simulink model "SBW_PID_controller"  (R2024b)
settings: Solver=FixedStepAuto  StartTime=0.0  StopTime=inf  FixedStep=0.001  RelTol=1e-3
model workspace (MAT data in the model file):
  th = 1
libraries: arduinolib x14, simulink x5, slpidlib x2
settings Model: ExtModeTrigDuration=2  Creator=masas  LastModifiedBy=masas
settings SolverCC: AutoInsertRateTranBlk=on
settings OptimizationCC: EnhancedBackFolding=on  PassReuseOutputArgsAs=Individual arguments  ZeroExternalMemoryAtStartup=off  ZeroInternalMemoryAtStartup=off  MaxStackSize=64  OptimizeBlockOrder=speed  DifferentSizesBufferReuse=on  OptimizationCustomize=off  EfficientTunableParamExpr=on
settings DebuggingCC: ParameterTunabilityLossMsg=error
settings HardwareCC: ProdBitPerInt=16  ProdBitPerPointer=16  ProdBitPerSizeT=16  ProdBitPerPtrDiffT=16  ProdLargestAtomicFloat=None  ProdWordSize=8  ProdHWDeviceType=Atmel->AVR  UseEmbeddedCoderFeatures=off
settings SFSimCC: MATLABDynamicMemAlloc=off
settings RTWCC: Description=Embedded Coder  SystemTargetFile=ert.tlc  HardwareBoard=Arduino Uno  TemplateMakefile=ert_default_tmf  Toolchain=Arduino AVR  BuildConfiguration=Faster Runs
settings CodeAppCC: ForceParamTrailComments=on  IgnoreCustomStorageClasses=off  OperatorAnnotations=on  SimulinkDataObjDesc=on  SFDataObjDesc=on  InsertBlockDesc=on
settings ERTTargetCC: SupportContinuousTime=on  SupportNonInlinedSFcns=on  SupportVariableSizeSignals=on  ExtModeTransport=3  ExtModeStaticAlloc=on  ExtModeAutomaticAllocSize=off  ExtModeStaticAllocSize=250  ExtModeMexFile=ext_xcp  ExtModeIntrfLevel=Level2 - Open  InlinedParameterPlacement=Hierarchical

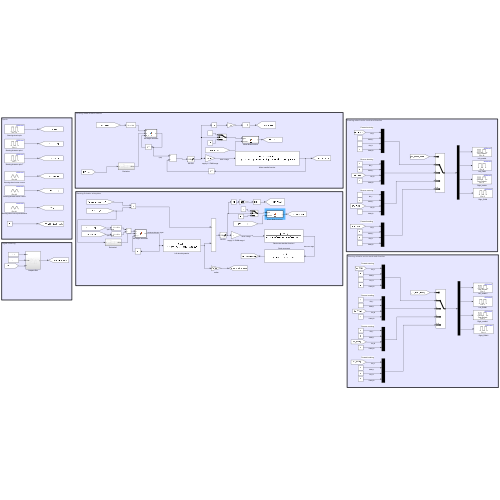
[thumbnail: Simulink's stored preview of the top-level diagram]
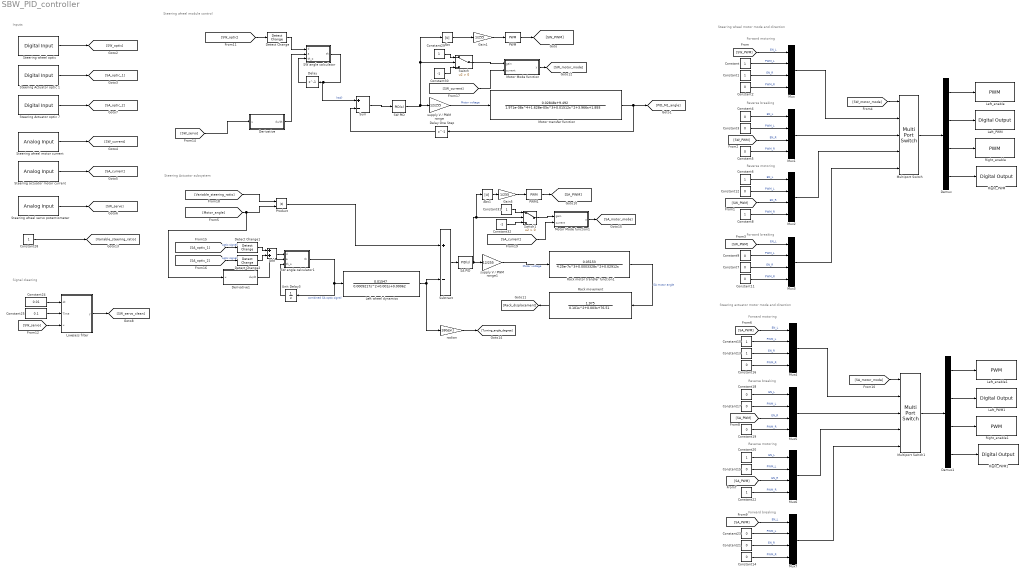
== system SBW_PID_controller ==
  note: Steering Actuator subsystem
  note: Signal cleaning
  note: Inputs
  note: Steering wheel module control
  note: Forward motoring
  note: Steering wheel motor mode and direction
  note: Reverse breaking
  note: Reverse motoring
  note: Forward breaking
  note: Forward breaking
  note: Reverse motoring
  note: Steering actuator motor mode and direction
  note: Forward motoring
  note: Reverse breaking
  Abs : Abs  SaturateOnIntegerOverflow=off
  Abs1 : Abs  SaturateOnIntegerOverflow=off
  Add : Sum
  Constant{,1,6,8,10,13,20,22,28..29,31} (11 alike) : Constant
  Constant{2..5,7,9,11..12,14..19,21,23} (16 alike) : Constant  Value=0
  Constant24 : Constant  Value=0.01
  Constant25 : Constant  Value=0.1
  Constant30 : Constant  Value=-1
  Constant32 : Constant  Value=-1
  Delay : Delay  DelayLength=1
  Delay One Step : Delay  DelayLength=1
  Demux : Demux
  Demux1 : Demux
  Derivative : Subsystem
  Derivative1 : Subsystem
  Detect Change : simulink/Logic and Bit Operations/Detect Change  vinit=0  OutDataTypeStr=boolean
  Detect Change1 : simulink/Logic and Bit Operations/Detect Change  vinit=0  OutDataTypeStr=boolean
  Detect Change2 : simulink/Logic and Bit Operations/Detect Change  vinit=0  OutDataTypeStr=boolean
  Gain1 : Gain  Gain=1/255
  Gain5 : Gain  Gain=1/255
  Left wheel dynamics : TransferFcn  Numerator=[0.01547]  Denominator=[0.0009217 0.001 0.00062]
  Left_PWM : arduinolib/Digital Output  pinNumber=8  Direction=output  blockPlatform=arduino
      settings: SourceProductName=Common
  Left_PWM1 : arduinolib/Digital Output  pinNumber=3  Direction=output  blockPlatform=arduino
      settings: SourceProductName=Common
  Left_enable : arduinolib/PWM  pinNumber=10  frequencyType=Default  desiredFrequency=490.2  achievableFrequency=490.2
      settings: SourceProductName=Common
  Left_enable1 : arduinolib/PWM  pinNumber=5  frequencyType=Default  desiredFrequency=490.2  achievableFrequency=490.2
      settings: SourceProductName=Common
  Lowpass filter : Subsystem
  Motor Mode function : MATLAB Function  TreatAsAtomicUnit=on
  Motor Mode function1 : MATLAB Function  TreatAsAtomicUnit=on
  Motor transfer function : TransferFcn  Numerator=[0.02848 9.492]  Denominator=|
      | [1.971e-08 1.628e-05 0.01512  3.966 1.893
      |  ]
  Multiport Switch : MultiPortSwitch  Inputs=4  SaturateOnIntegerOverflow=off  InputSameDT=off
  Multiport Switch1 : MultiPortSwitch  Inputs=4  SaturateOnIntegerOverflow=off  InputSameDT=off
  Mux{,1..7} (8 alike) : Mux
  PWM : simulink/Discontinuities/PWM  DisableCoverage=on  Period=0.01  InitialDelay=0  DisallowZeroDutyCycle=off  RunAtFixedTimeIntervals=on  SampleTime=0.1
  PWM1 : simulink/Discontinuities/PWM  DisableCoverage=on  Period=0.01  InitialDelay=0  DisallowZeroDutyCycle=off  RunAtFixedTimeIntervals=on  SampleTime=0.1
  Product : Product
  Rack motor transfer function1 : TransferFcn  Numerator=[0.05153]  Denominator=[4.25e-7 0.0003328 0.02912 0]
  Rack movement : TransferFcn  Numerator=[1.975]  Denominator=[0.101 0.003 76.51]
  Right_PWM : arduinolib/Digital Output  pinNumber=9  Direction=output  blockPlatform=arduino
      settings: SourceProductName=Common
  Right_PWM1 : arduinolib/Digital Output  pinNumber=4  Direction=output  blockPlatform=arduino
      settings: SourceProductName=Common
  Right_enable : arduinolib/PWM  pinNumber=11  frequencyType=Default  desiredFrequency=490.2  achievableFrequency=490.2
      settings: SourceProductName=Common
  Right_enable1 : arduinolib/PWM  pinNumber=6  frequencyType=Default  desiredFrequency=490.2  achievableFrequency=490.2
      settings: SourceProductName=Common
  "SA PID " : slpidlib/PID Controller  Controller=PID  Form=Parallel  TimeDomain=Continuous-time  UseExternalTs=off  SampleTime=-1  IntegratorMethod=Forward Euler  FilterMethod=Forward Euler  ControllerParametersSource=internal  P=6.187  I=0.03716  UseKiTs=off  D=19.07  UseExternalDerivativeSource=off  N=7.338  UseFilter=on  TunerSelectOption=Transfer Function Based (PID Tuner App)  InitialConditionSource=internal  InitialConditionForIntegrator=0  InitialConditionForFilter=0  DifferentiatorICPrevScaledInput=0  ExternalReset=none  TrackingMode=off  Kt=1  LimitOutput=on  SatLimitsSource=internal  UpperSaturationLimit=255  LowerSaturationLimit=-255  LinearizeAsGain=on  AntiWindupMode=none  Kb=1  LimitIntegrator=off  UpperIntegratorSaturationLimit=inf  LowerIntegratorSaturationLimit=-inf  POutMin=[]  POutMax=[]  IOutMin=[]  IOutMax=[]  DOutMin=[]  DOutMax=[]  NOutMin=[]  NOutMax=[]  SumOutMin=[]  SumOutMax=[]  SaturationOutMin=[]  SaturationOutMax=[]  PParamMin=[]  PParamMax=[]  IParamMin=[]  IParamMax=[]  DParamMin=[]  DParamMax=[]  NParamMin=[]  NParamMax=[]  KbParamMin=[]  KbParamMax=[]  KtParamMin=[]  KtParamMax=[]  KbOutMin=[]  KbOutMax=[]  KtOutMin=[]  KtOutMax=[]  IntegratorOutMin=[]  IntegratorOutMax=[]  FilterOutMin=[]  FilterOutMax=[]  SumI1OutMin=[]  SumI1OutMax=[]  SumI2OutMin=[]  SumI2OutMax=[]  SumI3OutMin=[]  SumI3OutMax=[]  SumI4OutMin=[]  SumI4OutMax=[]  SumDOutMin=[]  SumDOutMax=[]  DifferentiatorOutMin=[]  DifferentiatorOutMax=[]  FilterDiffOutCoefMin=[]  FilterDiffOutCoefMax=[]  ReciprocalOutMin=[]  ReciprocalOutMax=[]  SumDenOutMin=[]  SumDenOutMax=[]  SumNumOutMin=[]  SumNumOutMax=[]  DivideOutMin=[]  DivideOutMax=[]  UdiffTsProdOutMin=[]  UdiffTsProdOutMax=[]  NTsProdOutMin=[]  NTsProdOutMax=[]  UintegralTsProdOutMin=[]  UintegralTsProdOutMax=[]  UngainTsProdOutMin=[]  UngainTsProdOutMax=[]  ClampingZeroOutDataTypeStr=Inherit: Inherit via back propagation  ClampingZeroOutMin=[]  ClampingZeroOutMax=[]  FilterDenConstantOutDataTypeStr=Inherit: Inherit via back propagation  FilterDenConstantOutMin=[]  FilterDenConstantOutMax=[]  PCopyOutDataTypeStr=Inherit: Inherit via back propagation  PCopyOutMin=[]  PCopyOutMax=[]  NCopyOutDataTypeStr=Inherit: Inherit via back propagation  NCopyOutMin=[]  NCopyOutMax=[]  IntegratorContinuousStateAttributes=''  IntegratorStateMustResolveToSignalObject=off  IntegratorRTWStateStorageClass=Auto  FilterContinuousStateAttributes=''  FilterStateMustResolveToSignalObject=off  FilterRTWStateStorageClass=Auto  ParallelPVariant=InternalParameters  IdealPVariant=Disabled  IVariant=InternalParameters  DVariant=InternalParameters  IntegratorVariant=Continuous  SatVariant=Enabled  AWVariant=Passthrough  PCopyVariant=Disabled  TRVariant=Disabled  FdbkBlocksVariant=Forward  IdealPFdbkVariant=Disabled  SatFdbkVariant=Disabled  DerivativeFilterVariant=ContFilter  NVariant=InternalParameters  NCopyVariant=Disabled  FilterICVariant=InternalICsFilter  IntegratorICVariant=InternalICs  ExternalResetVariant=Disabled  TRSumVariant=Passthrough  SumFdbkVariant=Disabled  SumVariant=Sum_PID  TsampFilterVariant=InternalTs  TsampNgainVariant=Passthrough  TsampIntegralVariant=Disabled_SignalSpec  ExternalSaturationOutDataTypeStr=Inherit: Same as second input  DerivativeSourceVariant=ErrorSignal  PreIntVariant=InternalPreInt
  SW PID : slpidlib/PID Controller  Controller=PID  Form=Parallel  TimeDomain=Continuous-time  UseExternalTs=off  SampleTime=-1  IntegratorMethod=Forward Euler  FilterMethod=Forward Euler  ControllerParametersSource=internal  P=11.4731917903182  I=4.9291893088192  UseKiTs=off  D=3.34423646974898  UseExternalDerivativeSource=off  N=2.10860492250304  UseFilter=on  TunerSelectOption=Transfer Function Based (PID Tuner App)  InitialConditionSource=internal  InitialConditionForIntegrator=0  InitialConditionForFilter=0  DifferentiatorICPrevScaledInput=0  ExternalReset=none  TrackingMode=off  Kt=1  LimitOutput=on  SatLimitsSource=internal  UpperSaturationLimit=255  LowerSaturationLimit=-255  LinearizeAsGain=on  AntiWindupMode=clamping  Kb=1  LimitIntegrator=off  UpperIntegratorSaturationLimit=inf  LowerIntegratorSaturationLimit=-inf  POutMin=[]  POutMax=[]  IOutMin=[]  IOutMax=[]  DOutMin=[]  DOutMax=[]  NOutMin=[]  NOutMax=[]  SumOutMin=[]  SumOutMax=[]  SaturationOutMin=[]  SaturationOutMax=[]  PParamMin=[]  PParamMax=[]  IParamMin=[]  IParamMax=[]  DParamMin=[]  DParamMax=[]  NParamMin=[]  NParamMax=[]  KbParamMin=[]  KbParamMax=[]  KtParamMin=[]  KtParamMax=[]  KbOutMin=[]  KbOutMax=[]  KtOutMin=[]  KtOutMax=[]  IntegratorOutMin=[]  IntegratorOutMax=[]  FilterOutMin=[]  FilterOutMax=[]  SumI1OutMin=[]  SumI1OutMax=[]  SumI2OutMin=[]  SumI2OutMax=[]  SumI3OutMin=[]  SumI3OutMax=[]  SumI4OutMin=[]  SumI4OutMax=[]  SumDOutMin=[]  SumDOutMax=[]  DifferentiatorOutMin=[]  DifferentiatorOutMax=[]  FilterDiffOutCoefMin=[]  FilterDiffOutCoefMax=[]  ReciprocalOutMin=[]  ReciprocalOutMax=[]  SumDenOutMin=[]  SumDenOutMax=[]  SumNumOutMin=[]  SumNumOutMax=[]  DivideOutMin=[]  DivideOutMax=[]  UdiffTsProdOutMin=[]  UdiffTsProdOutMax=[]  NTsProdOutMin=[]  NTsProdOutMax=[]  UintegralTsProdOutMin=[]  UintegralTsProdOutMax=[]  UngainTsProdOutMin=[]  UngainTsProdOutMax=[]  ClampingZeroOutDataTypeStr=Inherit: Inherit via back propagation  ClampingZeroOutMin=[]  ClampingZeroOutMax=[]  FilterDenConstantOutDataTypeStr=Inherit: Inherit via back propagation  FilterDenConstantOutMin=[]  FilterDenConstantOutMax=[]  PCopyOutDataTypeStr=Inherit: Inherit via back propagation  PCopyOutMin=[]  PCopyOutMax=[]  NCopyOutDataTypeStr=Inherit: Inherit via back propagation  NCopyOutMin=[]  NCopyOutMax=[]  IntegratorContinuousStateAttributes=''  IntegratorStateMustResolveToSignalObject=off  IntegratorRTWStateStorageClass=Auto  FilterContinuousStateAttributes=''  FilterStateMustResolveToSignalObject=off  FilterRTWStateStorageClass=Auto  ParallelPVariant=InternalParameters  IdealPVariant=Disabled  IVariant=InternalParameters  DVariant=InternalParameters  IntegratorVariant=Continuous  SatVariant=Enabled  AWVariant=ContClampingParallel  PCopyVariant=Disabled  TRVariant=Disabled  FdbkBlocksVariant=Forward  IdealPFdbkVariant=Disabled  SatFdbkVariant=Disabled  DerivativeFilterVariant=ContFilter  NVariant=InternalParameters  NCopyVariant=Disabled  FilterICVariant=InternalICsFilter  IntegratorICVariant=InternalICs  ExternalResetVariant=Disabled  TRSumVariant=Passthrough  SumFdbkVariant=Disabled  SumVariant=Sum_PID  TsampFilterVariant=InternalTs  TsampNgainVariant=Passthrough  TsampIntegralVariant=Disabled_SignalSpec  ExternalSaturationOutDataTypeStr=Inherit: Same as second input  DerivativeSourceVariant=ErrorSignal  PreIntVariant=InternalPreInt
  SW angle calculator : MATLAB Function  TreatAsAtomicUnit=on
  SW angle calculator1 : MATLAB Function  TreatAsAtomicUnit=on
  Steering Actuator optic 1 : arduinolib/Digital Input  pinNumber=2  mode=Default  Direction=input  SampleTime=0.1  blockPlatform=arduino
      settings: SourceProductName=Common
  Steering Actuator optic 7 : arduinolib/Digital Input  pinNumber=7  mode=Default  Direction=input  SampleTime=0.1  blockPlatform=arduino
      settings: SourceProductName=Common
  Steering actuator motor current : arduinolib/Analog Input  pinNumber=3  ReadResultsOnly=off  ConversionTriggerSource=Software  ExternalTriggerType=uint32( 0 )  OutputDataType=uint16  EnableConversionCompleteNotify=off  EnableOuputStatus=off  SampleTime=-1  blockPlatform=arduino
      settings: SourceProductName=Common
  Steering wheel motor current : arduinolib/Analog Input  pinNumber=4  ReadResultsOnly=off  ConversionTriggerSource=Software  ExternalTriggerType=uint32( 0 )  OutputDataType=uint16  EnableConversionCompleteNotify=off  EnableOuputStatus=off  SampleTime=-1  blockPlatform=arduino
      settings: SourceProductName=Common
  Steering wheel optic : arduinolib/Digital Input  pinNumber=12  mode=Default  Direction=input  SampleTime=0.1  blockPlatform=arduino
      settings: SourceProductName=Common
  Steering wheel servo potentiometer : arduinolib/Analog Input  pinNumber=1  ReadResultsOnly=off  ConversionTriggerSource=Software  ExternalTriggerType=uint32( 0 )  OutputDataType=uint16  EnableConversionCompleteNotify=off  EnableOuputStatus=off  SampleTime=-1  blockPlatform=arduino
      settings: SourceProductName=Common
  Subtract : Sum  Inputs=+-
  Sum : Sum  Inputs=+-
  Switch : Switch  Criteria=u2 > Threshold  SaturateOnIntegerOverflow=off  InputSameDT=off
  Switch1 : Switch  Criteria=u2 > Threshold  SaturateOnIntegerOverflow=off  InputSameDT=off
  Unit Delay3 : UnitDelay  SampleTime=-1  HasFrameUpgradeWarning=on
  radian : Gain  Gain=180/pi()
  supply V / PWM range : Gain  Gain=12/255
  supply V / PWM range1 : Gain  Gain=12/255
  wires:
  [SW_optic] -> Detect Change/1
  Detect Change/1 -> SW angle calculator/1(d)
  Derivative/1(du/dt) -> SW angle calculator/2(a)
  SW angle calculator/1(th) -> Sum/1, Delay/1  "(rad)"
  [SW_PWM] -> Mux/1  "EN_L"
  Constant/1 -> Mux/2  "PWM_L"
  Constant1/1 -> Mux/3  "EN_R"
  Constant2/1 -> Mux/4  "PWM_R"
  Constant3/1 -> Mux1/2  "PWM_L"
  Constant4/1 -> Mux1/1  "EN_L"
  [SW_PWM] -> Mux1/3  "EN_R"
  Constant5/1 -> Mux1/4  "PWM_R"
  [SW_PWM] -> Mux2/3  "EN_R"
  [SW_PWM] -> Mux3/1  "EN_L"
  Constant9/1 -> Mux3/2  "PWM_L"
  Constant12/1 -> Mux2/2  "PWM_L"
  Constant6/1 -> Mux2/1  "EN_L"
  Constant7/1 -> Mux3/3  "EN_R"
  Constant11/1 -> Mux3/4  "PWM_R"
  Constant8/1 -> Mux2/4  "PWM_R"
  Mux3/1 -> Multiport Switch/5
  Mux2/1 -> Multiport Switch/4
  Mux1/1 -> Multiport Switch/3
  Mux/1 -> Multiport Switch/2
  [SW_motor_mode] -> Multiport Switch/1
  Multiport Switch/1 -> Demux/1
  Demux/4 -> Right_PWM/1
  Demux/3 -> Right_enable/1
  Demux/2 -> Left_PWM/1
  Demux/1 -> Left_enable/1
  Delay/1 -> SW angle calculator/3(th_o)
  Steering wheel optic/1 -> [SW_optic]
  [SA_PWM] -> Mux4/1  "EN_L"
  [SA_PWM] -> Mux6/3  "EN_R"
  Mux5/1 -> Multiport Switch1/3
  Constant15/1 -> Mux6/2  "PWM_L"
  Constant21/1 -> Mux7/3  "EN_R"
  Constant20/1 -> Mux6/1  "EN_L"
  Demux1/1 -> Left_enable1/1
  Constant13/1 -> Mux4/3  "EN_R"
  Demux1/3 -> Right_enable1/1
  Mux4/1 -> Multiport Switch1/2
  Constant19/1 -> Mux5/4  "PWM_R"
  Constant18/1 -> Mux5/1  "EN_L"
  Constant17/1 -> Mux5/2  "PWM_L"
  [SA_PWM] -> Mux5/3  "EN_R"
  Constant16/1 -> Mux4/4  "PWM_R"
  Constant14/1 -> Mux7/4  "PWM_R"
  Constant22/1 -> Mux6/4  "PWM_R"
  Demux1/4 -> Right_PWM1/1
  Constant10/1 -> Mux4/2  "PWM_L"
  Mux7/1 -> Multiport Switch1/5
  Multiport Switch1/1 -> Demux1/1
  [SA_PWM] -> Mux7/1  "EN_L"
  Mux6/1 -> Multiport Switch1/4
  [SA_motor_mode] -> Multiport Switch1/1
  Demux1/2 -> Left_PWM1/1
  Constant23/1 -> Mux7/2  "PWM_L"
  Steering Actuator optic 1/1 -> [SA_optic_1]
  Steering wheel motor current/1 -> [SW_current]
  Steering actuator motor current/1 -> [SA_current]
  Steering wheel servo potentiometer/1 -> [SW_servo]
  Lowpass filter/1(y) -> [SW_servo_clean]
  Constant25/1 -> Lowpass filter/2(Time)
  [SW_servo] -> Lowpass filter/3(u)
  Constant24/1 -> Lowpass filter/1(dt)
  [SW_servo] -> Derivative/1(u)
  [Motor_angle] -> Derivative1/1(u), Product/2
  Product/1 -> Subtract/1
  [Variable_steering_ratio] -> Product/1
  Constant28/1 -> [Variable_steering_ratio]
  Steering Actuator optic 7/1 -> [SA_optic_2]
  PWM/1 -> [SW_PWM]
  Sum/1 -> SW PID/1
  Motor transfer function/1 -> [PID_M1_angle], Delay One Step/1
  SW PID/1 -> Switch/2, Abs/1, supply V / PWM range/1
  Gain1/1 -> PWM/1
  Abs/1 -> Gain1/1
  supply V / PWM range/1 -> Motor transfer function/1  "Motor voltage"
  Delay One Step/1 -> Sum/2
  Detect Change2/1 -> Add/2
  Detect Change1/1 -> Add/1
  Unit Delay3/1 -> SW angle calculator1/3(th_o)
  SW angle calculator1/1(th) -> Unit Delay3/1, Left wheel dynamics/1  "combined SA optic signal"
  [SA_optic_2] -> Detect Change2/1  "optic signal"
  [SA_optic_1] -> Detect Change1/1  "optic signal"
  Rack movement/1 -> [Rack_displacement]
  Gain5/1 -> PWM1/1
  supply V / PWM range1/1 -> Rack motor transfer function1/1  "Motor voltage"
  Rack motor transfer function1/1 -> Rack movement/1  "SA motor angle"
  PWM1/1 -> [SA_PWM]
  Subtract/1 -> "SA PID "/1
  Abs1/1 -> Gain5/1
  radian/1 -> [Turning_angle_degree]
  Left wheel dynamics/1 -> radian/1, Subtract/2
  Constant29/1 -> Switch/1
  Constant30/1 -> Switch/3
  [SW_current] -> Motor Mode function/2(current)
  Switch/1 -> Motor Mode function/1(gain)
  Motor Mode function/1(y) -> [SW_motor_mode]
  Motor Mode function1/1(y) -> [SA_motor_mode]
  Constant31/1 -> Switch1/1
  Constant32/1 -> Switch1/3
  Switch1/1 -> Motor Mode function1/1(gain)
  "SA PID "/1 -> supply V / PWM range1/1, Switch1/2, Abs1/1
  [SA_current] -> Motor Mode function1/2(current)
  Derivative1/1(du/dt) -> SW angle calculator1/2(a)
  Add/1 -> SW angle calculator1/1(d)

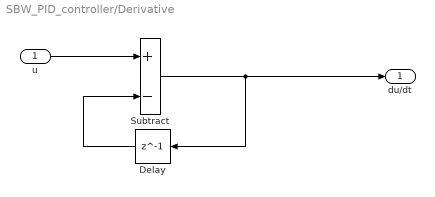
== system SBW_PID_controller/Derivative ==
  u : Inport
  Delay : Delay  DelayLength=1
  Subtract : Sum  Inputs=+-
  du/dt : Outport
  wires:
  Subtract/1 -> du/dt/1, Delay/1
  u/1 -> Subtract/1
  Delay/1 -> Subtract/2

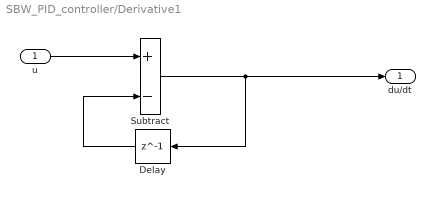
== system SBW_PID_controller/Derivative1 ==
  u : Inport
  Delay : Delay  DelayLength=1
  Subtract : Sum  Inputs=+-
  du/dt : Outport
  wires:
  Subtract/1 -> du/dt/1, Delay/1
  u/1 -> Subtract/1
  Delay/1 -> Subtract/2

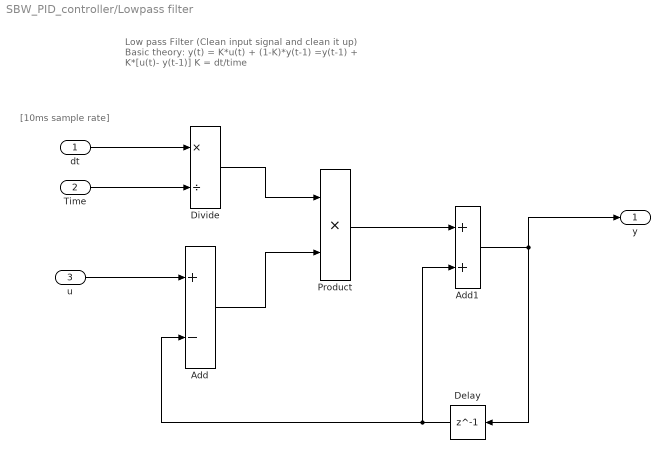
== system SBW_PID_controller/Lowpass filter ==
  note: [10ms sample rate]
  note: Low pass Filter (Clean input signal and clean it up)
      |
      | Basic theory: y(t) = K*u(t) + (1-K)*y(t-1)
      | 				=y(t-1) + K*[u(t)- y(t-1)]
      |
      | K = dt/time
  dt : Inport
  Time : Inport  Port=2
  u : Inport  Port=3
  Add : Sum  Inputs=+-
  Add1 : Sum
  Delay : Delay  DelayLength=1
  Divide : Product  Inputs=*/
  Product : Product
  y : Outport
  wires:
  dt/1 -> Divide/1
  Time/1 -> Divide/2
  u/1 -> Add/1
  Divide/1 -> Product/1
  Add/1 -> Product/2
  Add1/1 -> y/1, Delay/1
  Product/1 -> Add1/1
  Delay/1 -> Add/2, Add1/2

== matlab function SBW_PID_controller/SW angle calculator ==
  data: d input; th output; a input; th_o input
function th = fcn(d, a, th_o)

detector_slots = 200;

if ((d == true) && (a > 0))
    th = th_o + ((360/(2*detector_slots))* (pi/180));
elseif ((d == true) && (a < 0))
    th = th_o - ((360/(2*detector_slots))* (pi/180));
else 
    th = th_o;
end

== matlab function SBW_PID_controller/SW angle calculator1 ==
  data: d input; th output; a input; th_o input
function th = fcn(d, a, th_o)

detector_slots = 200;


if ((d == true) && (a > 0))
    th = th_o + ((360/(2*detector_slots))* (pi/180));
elseif ((d == true) && (a < 0))
    th = th_o - ((360/(2*detector_slots))* (pi/180));
else 
    th = th_o;
end

== matlab function SBW_PID_controller/Motor Mode function1 ==
  data: gain input; y output; current input
function y = fcn(gain, current)

if     ((current > 45) & (gain > 0)) %Forward motoring, but meeting resistance
    y = 2; %reverse braking
elseif ((current < 45) & (gain > 0)) %Forward motoring
    y = 1;
elseif ((current < 45) & (gain < 0)) %Reverse motoring
    y = 3;
elseif ((current > 45) & (gain < 0)) %Reverse motoring but meeting resistance
    y = 4;
else y =0;
end

== matlab function SBW_PID_controller/Motor Mode function ==
  data: gain input; y output; current input
function y = fcn(gain, current)

if     ((current > 45) & (gain > 0)) %Forward motoring, but meeting resistance
    y = 2; %reverse braking
elseif ((current < 45) & (gain > 0)) %Forward motoring
    y = 1;
elseif ((current < 45) & (gain < 0)) %Reverse motoring
    y = 3;
elseif ((current > 45) & (gain < 0)) %Reverse motoring but meeting resistance
    y = 4;
else y = 0;
end
